simulink model "case_2_lead_steady_then_slow"  (R2025b)
settings: Solver=VariableStepAuto  StartTime=0.0  StopTime=20.0  RelTol=1e-3
settings Model: Creator=sanborkl  LastModifiedBy=admin

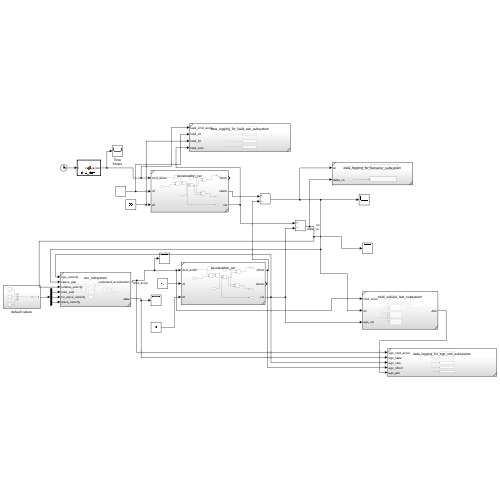
[thumbnail: Simulink's stored preview of the top-level diagram]
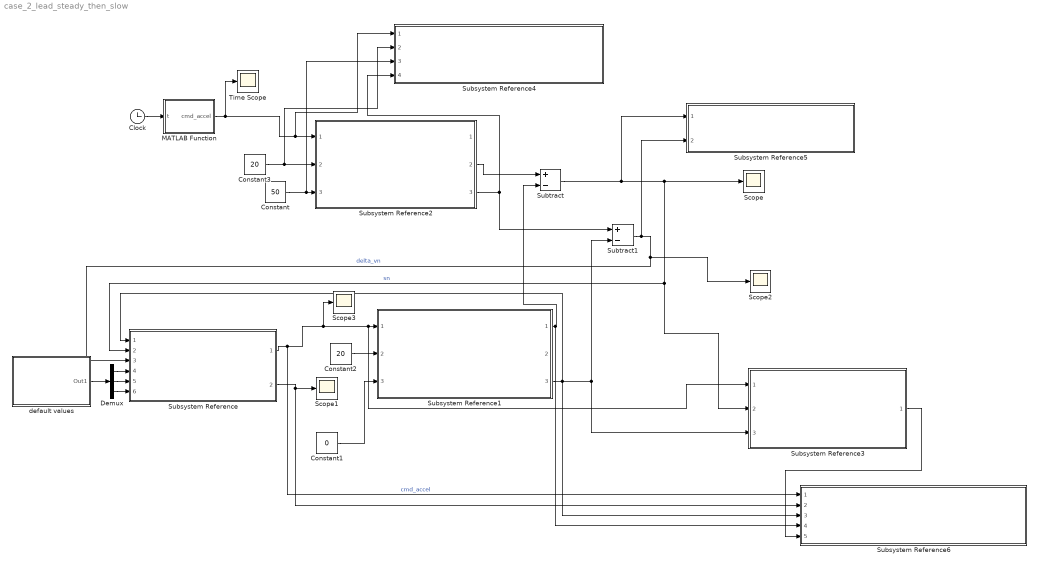
== system case_2_lead_steady_then_slow ==
  Clock : Clock
  Constant : Constant  Value=50
  Constant1 : Constant  Value=0
  Constant2 : Constant  Value=20
  Constant3 : Constant  Value=20
  Demux : Demux  Outputs=3
  MATLAB Function : MATLAB Function  TreatAsAtomicUnit=on
  Scope{,1..3} (4 alike) : Scope
      Scope settings: ActiveDisplayYMinimum=7.0577298305674168  ActiveDisplayYMaximum=50.060252241048069
      Scope1 settings: ActiveDisplayYMinimum=-1  ActiveDisplayYMaximum=1  DataLoggingVariableName=ScopeData2
      Scope2 settings: ActiveDisplayYMinimum=-2.373461653623723  ActiveDisplayYMaximum=2.9274500785935182  DataLoggingVariableName=ScopeData3
      Scope3 settings: ActiveDisplayYMinimum=-1.6601447210305178  ActiveDisplayYMaximum=1.8511271912256131  DataLoggingVariableName=ScopeData4
  Subsystem Reference : Subsystem  ReferencedSubsystem=acc_subsystem
  Subsystem Reference1 : Subsystem  ReferencedSubsystem=acceleration_car
  Subsystem Reference2 : Subsystem  ReferencedSubsystem=acceleration_car
  Subsystem Reference3 : Subsystem  ReferencedSubsystem=multi_vehicle_test_subsystem
  Subsystem Reference4 : Subsystem  ReferencedSubsystem=data_logging_for_lead_veh_subsystem
  Subsystem Reference5 : Subsystem  ReferencedSubsystem=data_logging_for_behavior_subsystem
  Subsystem Reference6 : Subsystem  ReferencedSubsystem=data_logging_for_ego_veh_subsystem
  Subtract : Sum  Inputs=+-
  Subtract1 : Sum  Inputs=+-
  Time Scope : Scope
      settings: TimeUnits=Metric (based on Time Span)  ActiveDisplayYMinimum=-1.0326734875444841  ActiveDisplayYMaximum=0.21732651245551637  YLabel=Amplitude
  default values : Subsystem
  wires:
  Subsystem Reference2/2 -> Subtract/1
  Subtract/1 -> Subsystem Reference5/1, Subsystem Reference3/2, Subsystem Reference/2, Scope/1  "sn"
  Subtract1/1 -> Subsystem Reference5/2, Subsystem Reference/3, Scope2/1  "delta_vn"
  Constant1/1 -> Subsystem Reference1/3
  Constant2/1 -> Subsystem Reference1/2
  Clock/1 -> MATLAB Function/1(t)
  Subsystem Reference1/1 -> Subsystem Reference6/4, Subtract/2
  Subsystem Reference/1 -> Subsystem Reference6/1, Scope3/1, Subsystem Reference3/1, Subsystem Reference1/1  "cmd_accel"
  Subsystem Reference/2 -> Subsystem Reference6/2, Scope1/1
  Subsystem Reference1/3 -> Subsystem Reference6/3, Subsystem Reference/1, Subsystem Reference3/3, Subtract1/2
  MATLAB Function/1(cmd_accel) -> Subsystem Reference2/1, Subsystem Reference4/1, Time Scope/1
  Constant3/1 -> Subsystem Reference2/2, Subsystem Reference4/2
  Constant/1 -> Subsystem Reference4/3, Subsystem Reference2/3
  Subsystem Reference2/3 -> Subsystem Reference4/4, Subtract1/1
  Subsystem Reference3/1 -> Subsystem Reference6/5
  Demux/1 -> Subsystem Reference/4
  default values/1(Out1) -> Demux/1
  Demux/2 -> Subsystem Reference/5
  Demux/3 -> Subsystem Reference/6

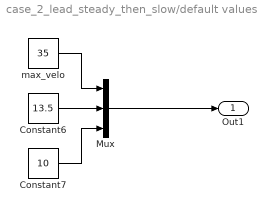
== system case_2_lead_steady_then_slow/default values ==
  Constant6 : Constant  Value=13.5
  Constant7 : Constant  Value=10
  Mux : Mux  Inputs=3
  max_velo : Constant  Value=35
  Out1 : Outport
  wires:
  Constant7/1 -> Mux/3
  Constant6/1 -> Mux/2
  max_velo/1 -> Mux/1
  Mux/1 -> Out1/1

== matlab function case_2_lead_steady_then_slow/MATLAB Function ==
  data: t input; cmd_accel output
function cmd_accel = slow_down(t)

if t < 4
    cmd_accel = 0;
else
    cmd_accel = -1;
end
